simulink model "embedded_with_transpose"  (Simulink 7.3)
settings: Solver=ode45  StartTime=0.0  StopTime=10.0  RelTol=1e-3
settings Model: Creator=Administrator  LastModifiedBy=hnine
settings OptimizationCC: InitFltsAndDblsToZero=on
settings DebuggingCC: SaveWithParameterizedLinksMsg=none

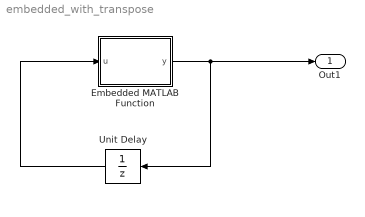
== system embedded_with_transpose ==
  Embedded MATLAB Function : Stateflow chart
  Unit Delay : UnitDelay  X0=[ 0 0 ; 0 0 ]
  Out1 : Outport  PortDimensions=[2 2]  DataType=single  OutDataType=sfix(16)  OutScaling=2^0  OutDataTypeStr=single
  wires:
  Embedded MATLAB Function/1(y) -> Unit Delay/1, Out1/1
  Unit Delay/1 -> Embedded MATLAB Function/1(u)

== matlab function Embedded MATLAB Function ==
  data: u input single size=[2 2]; y output single size=[2 2]
function y = fcn(u)
% This block supports the Embedded MATLAB subset.
% See the help menu for details. 

y = u' + [ 1 2 ; 3 4 ]'
